simulink model "Simulink_Lab2"  (R2016b)
settings: Solver=ode5  StartTime=0.0  StopTime=10.0  FixedStep=0.01  RelTol=1e-3  EnableMultiTasking=on
values from neighbouring files (symbols this model uses):
  C = 200    [Lab_2.m]
  K = 1000    [Lab_2.m]
  m = 10    [Lab_2.m]
settings Model: Creator=009768408  LastModifiedBy=Mac
settings DataIOCC: LimitDataPoints=on  SaveFormat=Array
settings OptimizationCC: LifeSpan=inf
settings DebuggingCC: SFUnexpectedBacktrackingDiag=warning  SFNoUnconditionalDefaultTransitionDiag=warning  SFExecutionAtInitializationDiag=none
settings HardwareCC: ProdBitPerPointer=32  ProdBitPerSizeT=32  ProdBitPerPtrDiffT=32  ProdLargestAtomicFloat=None  ProdIntDivRoundTo=Undefined  ProdEndianess=Unspecified  ProdWordSize=32  ProdHWDeviceType=32-bit Generic
settings ModelReferenceCC: PropagateSignalLabelsOutOfModel=off
settings GRTTargetCC: TargetLangStandard=C89/C90 (ANSI)  GeneratePreprocessorConditionals=Disable all
settings ConfigComp: CovMetricSettings=dw  CovHtmlReporting=on  CovSaveCumulativeToWorkspaceVar=on  CovSaveSingleToWorkspaceVar=on  CovExternalEMLEnable=off

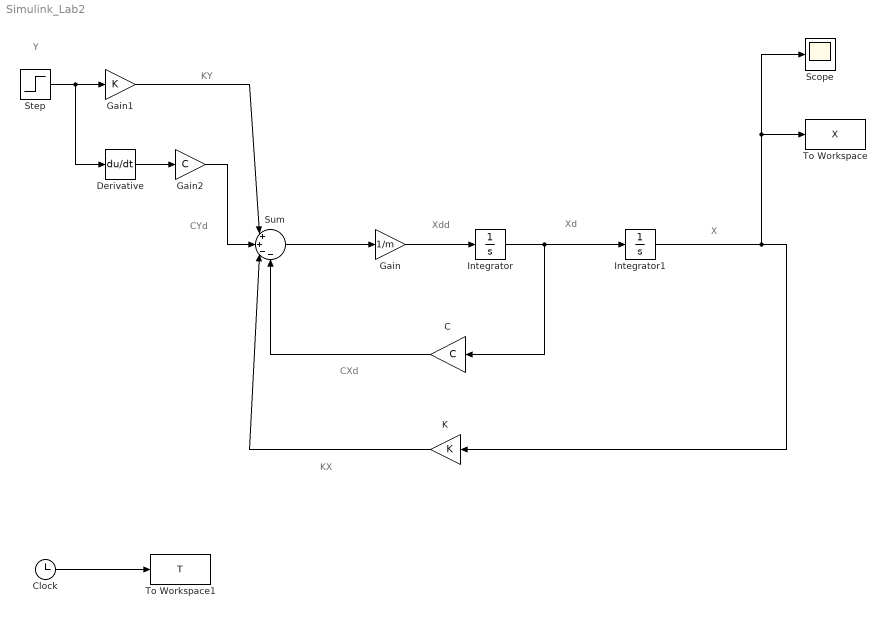
== system Simulink_Lab2 ==
  note: Y
  note: CYd
  note: KY
  note: CXd
  note: KX
  note: X
  note: Xd
  note: Xdd
  C : Gain  Gain=C
  Clock : Clock
  Derivative : Derivative
  Gain : Gain  Gain=1/m
  Gain1 : Gain  Gain=K
  Gain2 : Gain  Gain=C
  Integrator : Integrator
  Integrator1 : Integrator
  K : Gain  Gain=K
  Scope : Scope
  Step : Step  SampleTime=0
  Sum : Sum  Inputs=|++--
  To Workspace : ToWorkspace  VariableName=X  SampleTime=-1
  To Workspace1 : ToWorkspace  VariableName=T  SampleTime=-1
  wires:
  Sum/1 -> Gain/1
  Integrator1/1 -> Scope/1, To Workspace/1, K/1
  K/1 -> Sum/3
  Integrator/1 -> C/1, Integrator1/1
  Gain/1 -> Integrator/1
  C/1 -> Sum/4
  Step/1 -> Derivative/1, Gain1/1
  Derivative/1 -> Gain2/1
  Gain1/1 -> Sum/1
  Gain2/1 -> Sum/2
  Clock/1 -> To Workspace1/1
